simulink model "PuenteH_dcdc"  (R2024b)
settings: Solver=ode23s  StartTime=0.0  StopTime=Ts*nciclos  FixedStep=fixedstep  MaxStep=Ts/ssamples  RelTol=Auto  AbsTol=1e-3
InitFcn:
  | Ts=1/fs;
values from neighbouring files (symbols this model uses):
  fs = 10e3    (= 10000)    [Cuestion2.m]    (also in DatosBasePuenteH.m)
  ssamples = 200    [Cuestion2.m]    (also in DatosBasePuenteH.m)
  Vcont = 2*D - 1    [Cuestion2.m]    (also in DatosBasePuenteH.m = -0.6)
libraries: spsMultimeterLib x3, simulink x2, spsVoltageMeasurementLib x2, spsDCVoltageSourceLib x1, spsMeanLib x1, spsControlledVoltageSourceLib x1, spsCurrentMeasurementLib x1, spsSeriesRLCBranchLib x1, spsOnDelayLib x1, spsRMSLib x1, spsUniversalBridgeLib x1, sps_lib x1
settings Model: Creator=patrice  LastModifiedBy=Pablo
settings SolverCC: AutoScaleAbsTol=off  AlgebraicLoopSolver=TrustRegion
settings DataIOCC: SaveFormat=StructureWithTime  SignalLoggingSaveFormat=ModelDataLogs  ReturnWorkspaceOutputs=off  TimeSaveName=tiempo  SignalLoggingName=sigsOut
settings OptimizationCC: BlockReduction=off  BooleanDataType=off  ExpressionDepthLimit=2147483647  InitFltsAndDblsToZero=on  LifeSpan=inf
settings DebuggingCC: SaveWithParameterizedLinksMsg=none  UnderspecifiedInitializationDetection=Classic  MergeDetectMultiDrivingBlocksExec=none  SignalResolutionControl=TryResolveAllWithWarning  MultiTaskDSMMsg=warning  MultiTaskCondExecSysMsg=none  FcnCallInpInsideContextMsg=warning  StateNameClashWarn=warning  SFUnexpectedBacktrackingDiag=warning  SFNoUnconditionalDefaultTransitionDiag=warning  SFExecutionAtInitializationDiag=none  ArithmeticOperatorsInVariantConditions=warning
settings HardwareCC: ProdBitPerPointer=32  ProdBitPerSizeT=32  ProdBitPerPtrDiffT=32  ProdLargestAtomicFloat=None  ProdIntDivRoundTo=Undefined  ProdEndianess=Unspecified  ProdWordSize=32  ProdHWDeviceType=32-bit Generic  TargetUnknown=on
settings ModelReferenceCC: EnableRefExpFcnMdlSchedulingChecks=on  PropagateSignalLabelsOutOfModel=off
settings SFSimCC: SimUseLocalCustomCode=off  CustomCodeUndefinedFunction=UseInterfaceOnly
settings RTWCC: TemplateMakefile=grt_unix.tmf  RTWUseLocalCustomCode=off  GPUComputeCapability=3.5  DLArmComputeVersion=19.05
settings CodeAppCC: StateflowObjectComments=on
settings GRTTargetCC: TargetFcnLib=ansi_tfl_tmw.mat  TargetLangStandard=C89/C90 (ANSI)  CombineOutputUpdateFcns=off  GRTInterface=on
settings ConfigComp: CovMetricSettings=dw  CovSaveCumulativeToWorkspaceVar=on  CovSaveSingleToWorkspaceVar=on  CovExternalEMLEnable=off
settings SimscapeCC: SimscapeNormalizeSystem=off

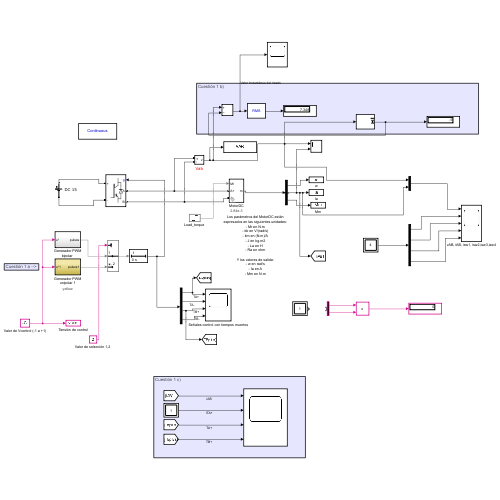
[thumbnail: Simulink's stored preview of the top-level diagram]
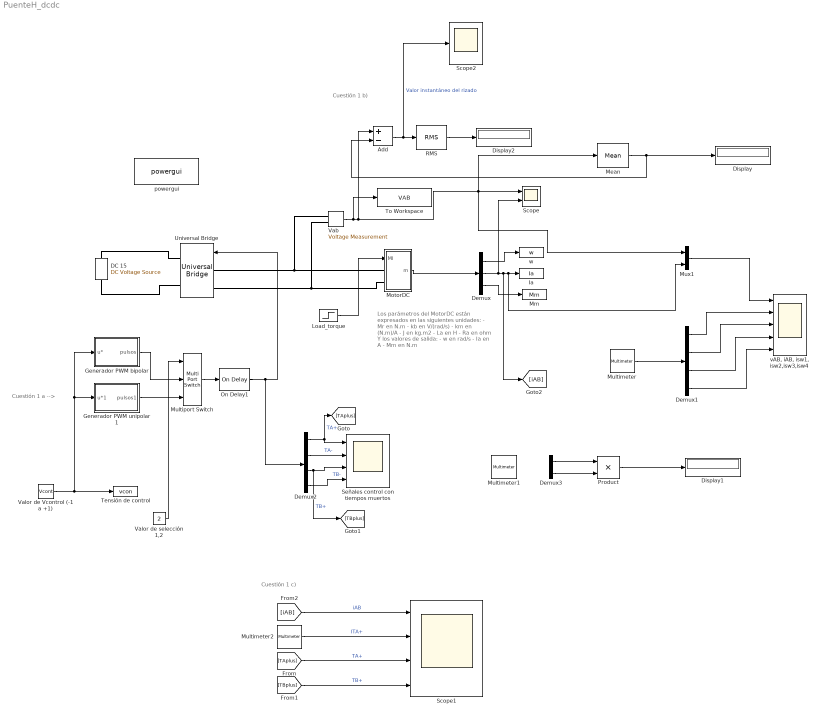
== system PuenteH_dcdc ==
  note: Cuestión 1 a -->
  note: Cuestión 1 b)
  note: Cuestión 1 c)
  note: Los parámetros del MotorDC están
      | expresados en las siguientes unidades:
      | - Mr en N.m
      | - kb en V/(rad/s)
      | - km en (N.m)/A
      | - J en kg.m2
      | - La en H
      | - Ra en ohm
      |
      | Y los valores de salida:
      | - w en rad/s
      | - Ia en A
      | - Mm en N.m
  Add : Sum  Inputs=+-
  DC 15 : spsDCVoltageSourceLib/DC Voltage Source  Amplitude=15  Measurements=Voltage
  Demux : Demux  Outputs=3
      settings: DisplayOption=none
  Demux1 : Demux
  Demux2 : Demux
  Demux3 : Demux  Outputs=2
  Display : Display
  Display1 : Display
  Display2 : Display
  "Generador PWM bipolar " : Subsystem
  Generador PWM unipolar 1 : Subsystem
      settings: AttributesFormatString=%<BackgroundColor>
  Ia : ToWorkspace  VariableName=Ia  SampleTime=-1
  "Load_torque " : Step  Time=0.12  After=0.02  SampleTime=0
  Mean : spsMeanLib/Mean  Freq=fs  Vinit=0  Ts=0
  Mm : ToWorkspace  VariableName=Mm  SampleTime=-1
  MotorDC : Subsystem  mask(Motor DC de imán permanente){Mr=2.84e-3, kb=35.1e-3, km=35.1e-3, J=43e-7, La=0.55e-3, Ra=4.09}
      mask prompts: Mr "Par de pérdidas (Mr)"; kb "Constante de velocidad (kb)"; km "Constante de par (km)"; J "Coeficiente de inercia (J)"; La "Inductancia de armadura (La)"; Ra "Resistencia de armadura (Ra)"
      settings: AttributesFormatString=%<Mr>
  Multimeter : spsMultimeterLib/Multimeter  L=11  sel=[8 9 10 11]  yselected={}  Gain=[1 1 1 1]  OutputType=Complex  PlotAtSimulationStop=off  PhasorSimulation=off
  Multimeter1 : spsMultimeterLib/Multimeter  L=11  sel=7  yselected={}  Gain=1  OutputType=Complex  PlotAtSimulationStop=off  PhasorSimulation=off
  Multimeter2 : spsMultimeterLib/Multimeter  L=11  sel=8  yselected={}  Gain=1  OutputType=Complex  PlotAtSimulationStop=off  PhasorSimulation=off
  Multiport Switch : MultiPortSwitch  Inputs=2  SaturateOnIntegerOverflow=off  InputSameDT=off
  Mux1 : Mux  Inputs=2
  On Delay1 : spsOnDelayLib/On Delay  DelayType=On delay  delay=Tmuertos  ic=0  Ts=0
  Product : Product
  RMS : spsRMSLib/RMS  TrueRMS=on  Freq=fs  RMSInit=120  Ts=0
  Scope : Scope  NumInputPorts=2
  Scope1 : Scope  NumInputPorts=4
  Scope2 : Scope
  Señales control con tiempos muertos : Scope  NumInputPorts=4
  Tensión de control : ToWorkspace  VariableName=vcon  SampleTime=-1
  To Workspace : ToWorkspace  VariableName=VAB  SaveFormat=Structure With Time  SampleTime=-1
  Universal Bridge : spsUniversalBridgeLib/Universal Bridge  Arms=2  SnubberResistance=1e5  SnubberCapacitance=inf  Device=IGBT / Diodes  Ron=1e-3  Lon=0  ForwardVoltages="[  0  0  ]"  ForwardVoltage=0  GTOparameters=[ 10e-6 , 20e-6 ]  IGBTparameters=[ 1e-6 , 2e-6 ]  Measurements=All voltages and currents  Measurements_2=None  converterType=Rectifier
  Vab : spsVoltageMeasurementLib/Voltage Measurement  PhasorSimulation=off  OutputType=Complex  PSBequivalent=0
  Valor de Vcontrol (-1 a +1) : Constant  Description=Aquí se ajusta el valor de la tensión de control, que tiene que estar entre -1 y +1 (valores de pico de la señal triangular)  Value=Vcont
  "Valor de selección 1,2 " : Constant  Value=2
  powergui : sps_lib/powergui  SimulationMode=Continuous  SampleTime=Ts/ssamples  frequency=60  Iterations=50  frequencyindice=0  Pbase=100e6  ErrMax=1e-4  UnitsV=kV  UnitsW=MW  buscounter=0  FunctionMessages=off  echomessages=off  EnableUseOfTLC=off  CurrentSourceSwitches=off  DisableSnubberDevices=off  DisableRonSwitches=off  DisableVfSwitches=off  DisplayEquations=off  AutomaticDiscreteSolvers=off  SolverType=Tustin/Backward Euler (TBE)  Interpol=off  ExternalGateDelay=off  methode=off  Ts=100  x0status=blocks  SPID=off  SwTol=0  HookPort=off  NonlinearTolerance=1e-4  nMaxIteration=100  ContinueOnMaxIteration=off  RestoreLinks=warning  ResistiveCurrentMeasurement=off  Frange=[0:2:500]  Ylog=off  Xlog=on  ShowGrid=off  save=off  variable=ZData  structure=OutputPuente  ZoomFFT=on  StartTime=0.1  cycles=2  DisplayStyle=4  fundamental=10e3  FreqAxis=off  MaxFrequency=20*10e3  frequencyindicesteady=1  RmsSteady=1  display=off
  "vAB, iAB, isw1, isw2,isw3,isw4" : Scope  NumInputPorts=5
  w : ToWorkspace  VariableName=w  SampleTime=-1
  wires:
  "Generador PWM bipolar "/1(pulsos) -> Multiport Switch/2
  "Valor de selección 1,2 "/1 -> Multiport Switch/1
  Valor de Vcontrol (-1 a +1)/1 -> Tensión de control/1, Generador PWM unipolar 1/1(u*1), "Generador PWM bipolar "/1(u*)
  MotorDC/1(m) -> Demux/1
  Demux/2 -> Scope/2, [iAB], Mux1/2, Ia/1
  Demux/3 -> Mm/1
  Demux/1 -> w/1
  "Load_torque "/1 -> MotorDC/1(Ml)
  Vab/1 -> To Workspace/1, Add/1, Mux1/1, Mean/1, Scope/1
  Mean/1 -> Add/2, Display/1
  Multimeter/1 -> Demux1/1
  Mux1/1 -> "vAB, iAB, isw1, isw2,isw3,isw4"/1
  Demux1/1 -> "vAB, iAB, isw1, isw2,isw3,isw4"/2
  Demux1/2 -> "vAB, iAB, isw1, isw2,isw3,isw4"/3
  Demux1/3 -> "vAB, iAB, isw1, isw2,isw3,isw4"/4
  Demux1/4 -> "vAB, iAB, isw1, isw2,isw3,isw4"/5
  On Delay1/1 -> Demux2/1, Universal Bridge/1
  Multiport Switch/1 -> On Delay1/1
  Demux2/1 -> [TAplus], Señales control con tiempos muertos/1  "TA+"
  Demux2/2 -> Señales control con tiempos muertos/2  "TA-"
  Demux2/3 -> Señales control con tiempos muertos/3, [TBplus]  "TB+"
  Demux2/4 -> Señales control con tiempos muertos/4  "TB-"
  Generador PWM unipolar 1/1(pulsos1) -> Multiport Switch/3
  Demux3/1 -> Product/1
  Demux3/2 -> Product/2
  Product/1 -> Display1/1
  [TAplus] -> Scope1/3  "TA+"
  [TBplus] -> Scope1/4  "TB+"
  Multimeter2/1 -> Scope1/2  "ITA+"
  [iAB] -> Scope1/1  "iAB"
  RMS/1 -> Display2/1
  Add/1 -> Scope2/1, RMS/1  "Valor instantáneo del rizado"
  connections:
  MotorDC/LConn1 -- Universal Bridge/LConn1 -- Vab/LConn1
  MotorDC/LConn2 -- Vab/LConn2 -- Universal Bridge/LConn2
  DC 15/LConn1 -- Universal Bridge/RConn2
  Universal Bridge/RConn1 -- DC 15/RConn1

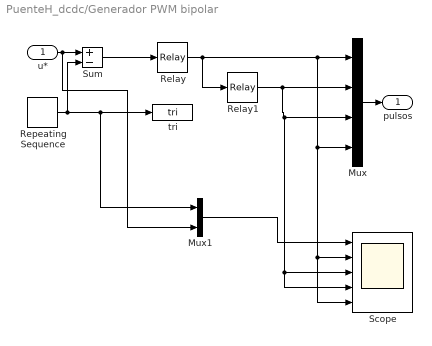
== system PuenteH_dcdc/Generador PWM bipolar  ==
  u* : Inport
  Mux : Mux
  Mux1 : Mux  Inputs=2
  Relay : Relay  OnSwitchValue=0.01  OffSwitchValue=-0.01
  Relay1 : Relay  OnSwitchValue=0.51  OffSwitchValue=0.49  OnOutputValue=0  OffOutputValue=1
  Repeating Sequence : simulink/Sources/Repeating Sequence  rep_seq_t="[0 Ts/2  Ts]"  rep_seq_y=[-1 1 -1]
  Scope : Scope  NumInputPorts=5
  Sum : Sum  Inputs=+-  InputSameDT=on  SaturateOnIntegerOverflow=on  OutDataTypeStr=Inherit: Same as first input
  tri : ToWorkspace  VariableName=tri  SampleTime=-1
  pulsos : Outport
  wires:
  Sum/1 -> Relay/1
  Repeating Sequence/1 -> Sum/2, Mux1/1, tri/1
  u*/1 -> Mux1/2, Sum/1
  Relay1/1 -> Mux/2, Scope/4, Scope/3, Mux/3
  Mux/1 -> pulsos/1
  Mux1/1 -> Scope/1
  Relay/1 -> Relay1/1, Mux/1, Scope/2, Scope/5, Mux/4

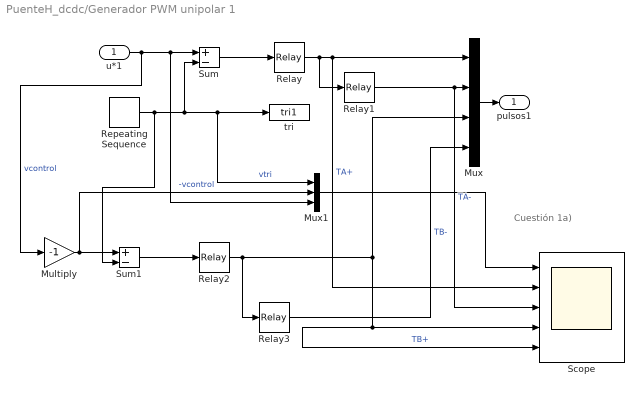
== system PuenteH_dcdc/Generador PWM unipolar 1 ==
  note: Cuestión 1a)
  u*1 : Inport
  Multiply : Gain  Gain=-1
  Mux : Mux
  Mux1 : Mux  Inputs=3
  Relay : Relay  OnSwitchValue=0.01  OffSwitchValue=-0.01
  Relay1 : Relay  OnSwitchValue=0.51  OffSwitchValue=0.49  OnOutputValue=0  OffOutputValue=1
  Relay2 : Relay  OnSwitchValue=0.01  OffSwitchValue=-0.01
  Relay3 : Relay  OnSwitchValue=0.51  OffSwitchValue=0.49  OnOutputValue=0  OffOutputValue=1
  Repeating Sequence : simulink/Sources/Repeating Sequence  rep_seq_t="[0 Ts/2  Ts]"  rep_seq_y=[-1 1 -1]
  Scope : Scope  NumInputPorts=5
  Sum : Sum  Inputs=+-  InputSameDT=on  SaturateOnIntegerOverflow=on  OutDataTypeStr=Inherit: Same as first input
  Sum1 : Sum  Inputs=+-  InputSameDT=on  SaturateOnIntegerOverflow=on  OutDataTypeStr=Inherit: Same as first input
  tri : ToWorkspace  VariableName=tri1  SampleTime=-1
  pulsos1 : Outport
  wires:
  Repeating Sequence/1 -> Sum1/2, Sum/2, Mux1/1, tri/1  "vtri"
  Mux/1 -> pulsos1/1
  u*1/1 -> Multiply/1, Mux1/3, Sum/1  "vcontrol"
  Sum/1 -> Relay/1
  Relay/1 -> Relay1/1, Mux/1, Scope/2  "TA+"
  Relay1/1 -> Scope/3, Mux/2  "TA-"
  Multiply/1 -> Mux1/2, Sum1/1  "-vcontrol"
  Sum1/1 -> Relay2/1
  Relay2/1 -> Relay3/1, Mux/3, Scope/5, Scope/4  "TB+"
  Relay3/1 -> Mux/4  "TB-"
  Mux1/1 -> Scope/1

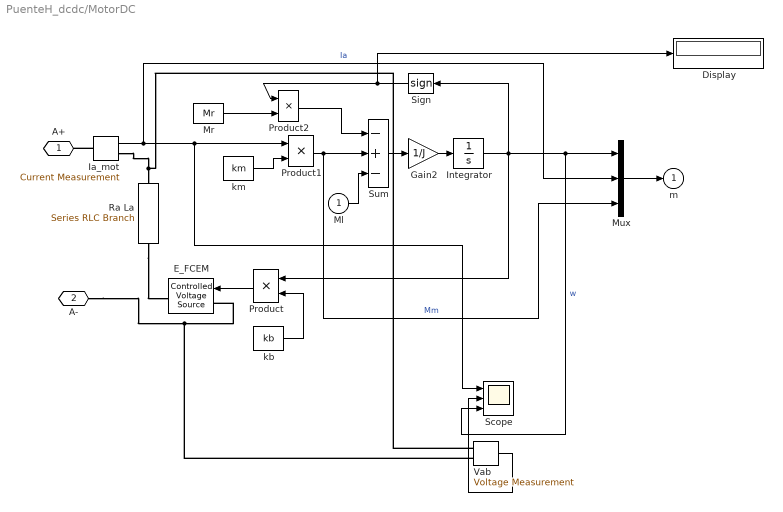
== system PuenteH_dcdc/MotorDC ==
  Ml : Inport
  Display : Display
  E_FCEM : spsControlledVoltageSourceLib/Controlled Voltage Source  Initialize=on  Source_Type=AC  Amplitude=0  Phase=0  Frequency=0  Measurements=None
  Gain2 : Gain  Gain=1/J  SaturateOnIntegerOverflow=on  OutDataTypeStr=Inherit: Same as input  ParamDataTypeStr=Inherit: Same as input
  Ia_mot : spsCurrentMeasurementLib/Current Measurement  PhasorSimulation=off  OutputType=Complex  PSBequivalent=0
  Integrator : Integrator  ZeroCross=off
  Mr : Constant  Value=Mr
  Mux : Mux  Inputs=3
  Product : Product  InputSameDT=on  SaturateOnIntegerOverflow=on  OutDataTypeStr=Inherit: Same as first input
  Product1 : Product  InputSameDT=on  SaturateOnIntegerOverflow=on  OutDataTypeStr=Inherit: Same as first input
  Product2 : Product  InputSameDT=on  SaturateOnIntegerOverflow=on  OutDataTypeStr=Inherit: Same as first input
  Ra La : spsSeriesRLCBranchLib/Series RLC Branch  LConnTagsString=__new0  RConnTagsString=__new0  BranchType=RLC  Resistance=Ra  Inductance=La  SetiL0=off  InitialCurrent=0  Capacitance=inf  Setx0=off  InitialVoltage=0  Measurements=None
  Scope : Scope  NumInputPorts=3
  Sign : Signum  ZeroCross=off
  Sum : Sum  Inputs=-+-  InputSameDT=on  SaturateOnIntegerOverflow=on  OutDataTypeStr=Inherit: Same as first input
  Vab : spsVoltageMeasurementLib/Voltage Measurement  PhasorSimulation=off  OutputType=Complex  PSBequivalent=0
  kb : Constant  Value=kb
  km : Constant  Value=km
  A+ : PMIOPort  Side=Left
  A- : PMIOPort  Port=2  Side=Left
  m : Outport  InitialOutput=0
  wires:
  km/1 -> Product1/2
  kb/1 -> Product/2
  Ia_mot/1 -> Mux/2, Scope/1, Product1/1  "Ia"
  Product2/1 -> Sum/1
  Sign/1 -> Display/1, Product2/1
  Sum/1 -> Gain2/1
  Gain2/1 -> Integrator/1
  Integrator/1 -> Sign/1, Scope/3, Mux/1, Product/1  "w"
  Product/1 -> E_FCEM/1
  Product1/1 -> Sum/2, Mux/3  "Mm"
  Mux/1 -> m/1
  Mr/1 -> Product2/2
  Ml/1 -> Sum/3
  Vab/1 -> Scope/2
  connections:
  Ia_mot/RConn1 -- Vab/LConn1 -- Ra La/LConn1
  Ra La/RConn1 -- E_FCEM/RConn1
  Ia_mot/LConn1 -- A+/RConn1
  A-/RConn1 -- Vab/LConn2 -- E_FCEM/LConn1
